simulink model "local"  (R2022a)
settings: Solver=VariableStepAuto  StartTime=0.0  StopTime=T_fin  FixedStep=0.0025  RelTol=1e-3
values from neighbouring files (symbols this model uses):
  A = A-B*k_leader    [project.m]
  Ad = [0 0 1 0 0 0; 1 0 0 0 0 0;0 1 0 0 0 0; 1 0 0 0 0 0; 0 0 0 0 0 0; 0 0 1 0 0 0]    [project.m]
  B = [0; -9.9453]    [project.m]
  C = [708.27 0]    [project.m]
  c = 5    [project.m]
  D_ = zeros(2,1)'    [project.m]
  F2 = place(A',-c*C',[-1 -2])'    [project.m]
  G = diag([1 0 0 0 1 0])    [project.m]
  K = inv(R)*B'*P    [project.m]
  L_leader = acker(A',C',[-1,-2])'    [project.m]
  X0 = [1/C(1) 1/800]'    [project.m]
settings Model: Creator=drurb  LastModifiedBy=Utente
settings DataIOCC: ReturnWorkspaceOutputs=off

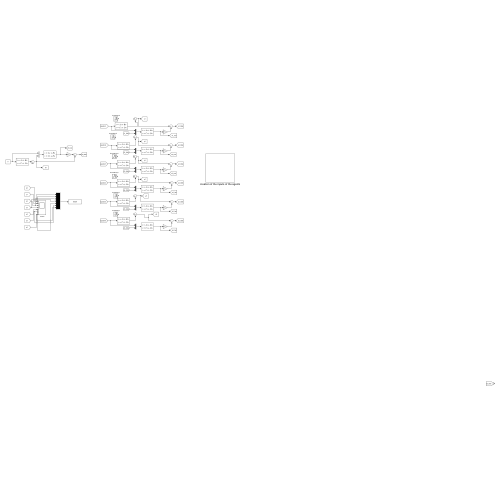
[thumbnail: Simulink's stored preview of the top-level diagram]
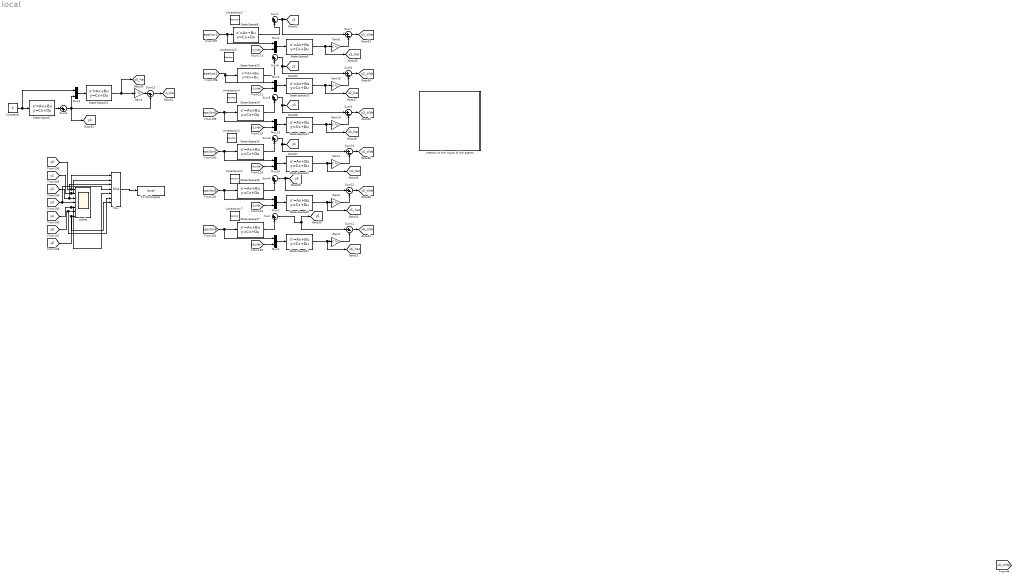
== system local ==
  Constant1 : Constant  Value=0
  Gain{1..5,13..14} (7 alike) : Gain  Gain=C  Multiplication=Matrix(K*u)
  Locale : Scope  NumInputPorts=7
  Mux : Mux  Inputs=7
  Mux{1..5,13..14} (7 alike) : Mux  Inputs=2
  State-Space{9..12,20..21} (6 alike) : StateSpace  A=A  B=[B*c*K -c*F2]  C=eye(2)  D=zeros(2,3)  InitialCondition=zeros(1,2)
  State-Space22 : StateSpace  A=A - L_leader*C  B=[B L_leader]  C=eye(2)  D=zeros(2,2)  InitialCondition=zeros(1,2)
  State-Space23 : StateSpace  A=A  B=B*c*K  C=C  D=D_  InitialCondition=[0 2/800]'
  State-Space24 : StateSpace  A=A  B=B*c*K  C=C  D=D_  InitialCondition=[-1/C(1) -1/800]
  State-Space25 : StateSpace  A=A  B=B*c*K  C=C  D=D_  InitialCondition=[3/C(1) -3/800]'
  State-Space26 : StateSpace  A=A  B=B*c*K  C=C  D=D_  InitialCondition=[2/C(1) 4/800]'
  State-Space27 : StateSpace  A=A  B=B*c*K  C=C  D=D_  InitialCondition=[-2/C(1) 0]'
  State-Space7 : StateSpace  A=A  B=B  C=C  D=0  InitialCondition=X0
  State-Space8 : StateSpace  A=A  B=B*c*K  C=C  D=D_  InitialCondition=[2/C(1) 1/800]'
  Sum{,1..6} (7 alike) : Sum  Inputs=|++
  Sum{7..12} (6 alike) : Sum  Inputs=|+-
  Sum13 : Sum  Inputs=|-+
  To Workspace : ToWorkspace  VariableName=local  SaveFormat=Timeseries  SampleTime=-1
  Uncertainty1 : RandomNumber  Mean=zeros(1,1)  Variance=0.1  Seed=1  SampleTime=0.1
  Uncertainty2 : RandomNumber  Seed=2  SampleTime=0.2
  Uncertainty3 : RandomNumber  Mean=zeros(1,1)  Variance=0.7  Seed=3  SampleTime=0.1
  Uncertainty4 : RandomNumber  Mean=zeros(1,1)  Variance=0.2  Seed=7  SampleTime=0.1
  Uncertainty5 : RandomNumber  Mean=zeros(1,1)  Variance=0.5  Seed=7  SampleTime=0.1
  Uncertainty7 : RandomNumber  Mean=zeros(1,1)  Variance=0.4  Seed=3  SampleTime=0.1
  creation of the inputs of the agents : Subsystem
  tag scope: x0_hat=global, x1_hat=global, x2_hat=global, x3_hat=global, x4_hat=global, x5_hat=global, x6_hat=global, y0=global, y0_tilde=global, y1=global, y1_tilde=global, y2=global, y2_tilde=global, y3=global, y3_tilde=global, y4=global, y4_tilde=global, y5=global, y5_tilde=global, y6=global, y6_tilde=global
  wires:
  State-Space11/1 -> [x3_hat], Gain14/1
  Gain1/1 -> Sum10/2
  [y1_tilde] -> Mux4/2
  Gain2/1 -> Sum11/2
  [epsilon4] -> State-Space25/1, Mux14/1
  Mux14/1 -> State-Space12/1
  Sum11/1 -> [y5_tilde]
  State-Space21/1 -> [x6_hat], Gain3/1
  Sum7/1 -> [y1_tilde]
  [y4_tilde] -> Mux14/2
  [epsilon2] -> State-Space23/1, Mux5/1
  Gain3/1 -> Sum12/2
  [epsilon5] -> State-Space26/1, Mux1/1
  State-Space9/1 -> Gain5/1, [x1_hat]
  Mux3/1 -> State-Space22/1
  [epsilon3] -> Mux13/1, State-Space24/1
  Sum12/1 -> [y6_tilde]
  [epsilon6] -> State-Space27/1, Mux2/1
  [epsilon1] -> Mux4/1, State-Space8/1
  Mux4/1 -> State-Space9/1
  [y5_tilde] -> Mux1/2
  [y3_tilde] -> Mux13/2
  Constant1/1 -> Mux3/1, State-Space7/1
  Sum10/1 -> [y4_tilde]
  [y3] -> Locale/4, Mux/4
  Mux2/1 -> State-Space21/1
  Gain4/1 -> Sum13/1
  Mux13/1 -> State-Space11/1
  Gain13/1 -> Sum8/2
  State-Space10/1 -> [x2_hat], Gain13/1
  Gain14/1 -> Sum9/2
  [y0] -> Mux/1, Locale/1
  [y1] -> Mux/2, Locale/2
  [y6] -> Mux/7, Locale/7
  [y6_tilde] -> Mux2/2
  Mux5/1 -> State-Space10/1
  State-Space20/1 -> [x5_hat], Gain2/1
  State-Space26/1 -> Sum4/2
  Mux1/1 -> State-Space20/1
  State-Space22/1 -> Gain4/1, [x0_hat]
  Sum9/1 -> [y3_tilde]
  Sum13/1 -> [y0_tilde]
  [y2_tilde] -> Mux5/2
  [y5] -> Locale/6, Mux/6
  State-Space12/1 -> [x4_hat], Gain1/1
  [y4] -> Mux/5, Locale/5
  Sum8/1 -> [y2_tilde]
  [y2] -> Locale/3, Mux/3
  Gain5/1 -> Sum7/2
  Mux/1 -> To Workspace/1
  State-Space27/1 -> Sum/2
  Sum/1 -> Sum12/1, [y6]
  Sum1/1 -> Sum7/1, [y1]
  State-Space8/1 -> Sum1/2
  State-Space7/1 -> Sum2/1
  Sum2/1 -> Sum13/2, [y0], Mux3/2
  State-Space25/1 -> Sum3/2
  Sum3/1 -> Sum10/1, [y4]
  Sum4/1 -> Sum11/1, [y5]
  Sum6/1 -> Sum8/1, [y2]
  State-Space23/1 -> Sum6/2
  Sum5/1 -> Sum9/1, [y3]
  State-Space24/1 -> Sum5/2

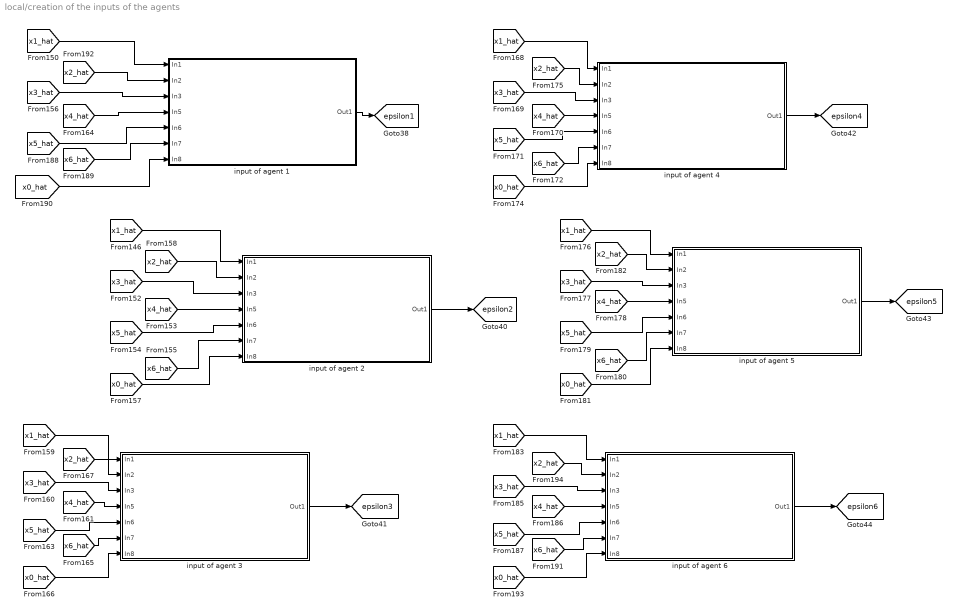
== system local/creation of the inputs of the agents ==
  input of agent 1 : Subsystem
  input of agent 2 : Subsystem
  input of agent 3 : Subsystem
  input of agent 4 : Subsystem
  input of agent 5 : Subsystem
  input of agent 6 : Subsystem
  tag scope: epsilon1=global, epsilon2=global, epsilon3=global, epsilon4=global, epsilon5=global, epsilon6=global
  wires:
  [x6_hat] -> input of agent 6/6(In7)
  input of agent 2/1(Out1) -> [epsilon2]
  [x0_hat] -> input of agent 3/7(In8)
  input of agent 6/1(Out1) -> [epsilon6]
  [x6_hat] -> input of agent 5/6(In7)
  [x2_hat] -> input of agent 5/2(In2)
  [x1_hat] -> input of agent 2/1(In1)
  [x1_hat] -> input of agent 4/1(In1)
  [x0_hat] -> input of agent 4/7(In8)
  [x5_hat] -> input of agent 1/5(In6)
  [x4_hat] -> input of agent 1/4(In5)
  [x4_hat] -> input of agent 5/4(In5)
  [x4_hat] -> input of agent 2/4(In5)
  input of agent 5/1(Out1) -> [epsilon5]
  [x3_hat] -> input of agent 6/3(In3)
  [x5_hat] -> input of agent 5/5(In6)
  [x5_hat] -> input of agent 3/5(In6)
  [x2_hat] -> input of agent 2/2(In2)
  [x4_hat] -> input of agent 6/4(In5)
  [x0_hat] -> input of agent 2/7(In8)
  [x5_hat] -> input of agent 6/5(In6)
  [x6_hat] -> input of agent 3/6(In7)
  [x1_hat] -> input of agent 5/1(In1)
  [x0_hat] -> input of agent 6/7(In8)
  [x3_hat] -> input of agent 1/3(In3)
  [x5_hat] -> input of agent 4/5(In6)
  [x3_hat] -> input of agent 3/3(In3)
  input of agent 4/1(Out1) -> [epsilon4]
  [x5_hat] -> input of agent 2/5(In6)
  [x1_hat] -> input of agent 1/1(In1)
  [x4_hat] -> input of agent 3/4(In5)
  [x4_hat] -> input of agent 4/4(In5)
  [x0_hat] -> input of agent 5/7(In8)
  [x1_hat] -> input of agent 6/1(In1)
  [x6_hat] -> input of agent 2/6(In7)
  [x2_hat] -> input of agent 6/2(In2)
  [x6_hat] -> input of agent 4/6(In7)
  [x2_hat] -> input of agent 1/2(In2)
  [x2_hat] -> input of agent 3/2(In2)
  [x3_hat] -> input of agent 4/3(In3)
  [x3_hat] -> input of agent 5/3(In3)
  [x0_hat] -> input of agent 1/7(In8)
  [x3_hat] -> input of agent 2/3(In3)
  [x1_hat] -> input of agent 3/1(In1)
  input of agent 3/1(Out1) -> [epsilon3]
  input of agent 1/1(Out1) -> [epsilon1]
  [x6_hat] -> input of agent 1/6(In7)
  [x2_hat] -> input of agent 4/2(In2)

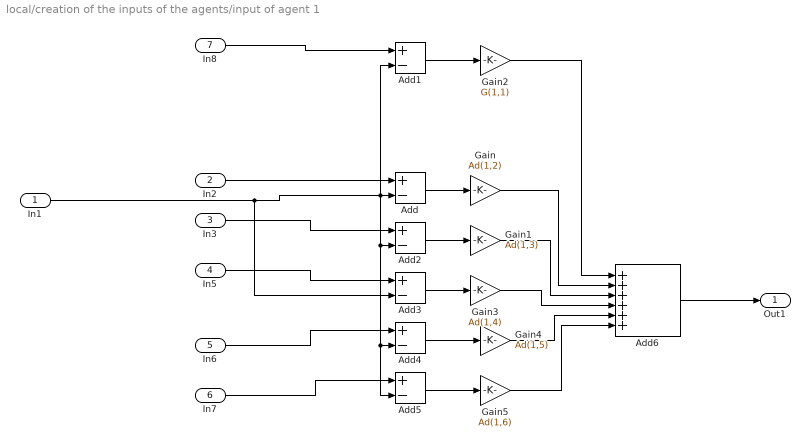
== system local/creation of the inputs of the agents/input of agent 1 ==
  In1 : Inport
  In2 : Inport  Port=2
  In3 : Inport  Port=3
  In5 : Inport  Port=4
  In6 : Inport  Port=5
  In7 : Inport  Port=6
  In8 : Inport  Port=7
  Add{,1..5} (6 alike) : Sum  Inputs=+-
  Add6 : Sum  Inputs=++++++
  Gain : Gain  Gain=Ad(1,2)
  Gain1 : Gain  Gain=Ad(1,3)
  Gain2 : Gain  Gain=G(1,1)
  Gain3 : Gain  Gain=Ad(1,4)
  Gain4 : Gain  Gain=Ad(1,5)
  Gain5 : Gain  Gain=Ad(1,6)
  Out1 : Outport
  wires:
  Add/1 -> Gain/1
  In1/1 -> Add3/2, Add5/2, Add4/2, Add2/2, Add/2, Add1/2
  In2/1 -> Add/1
  In8/1 -> Add1/1
  Add2/1 -> Gain1/1
  Add3/1 -> Gain3/1
  Add4/1 -> Gain4/1
  Add5/1 -> Gain5/1
  In3/1 -> Add2/1
  In5/1 -> Add3/1
  In6/1 -> Add4/1
  In7/1 -> Add5/1
  Gain/1 -> Add6/2
  Gain1/1 -> Add6/3
  Gain3/1 -> Add6/4
  Gain4/1 -> Add6/5
  Gain5/1 -> Add6/6
  Add1/1 -> Gain2/1
  Gain2/1 -> Add6/1
  Add6/1 -> Out1/1

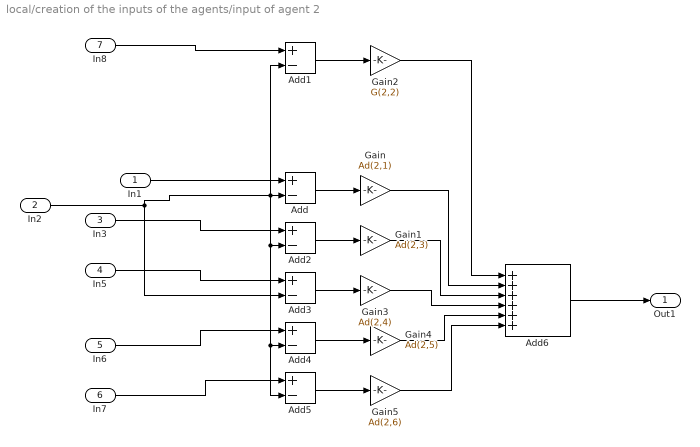
== system local/creation of the inputs of the agents/input of agent 2 ==
  In1 : Inport
  In2 : Inport  Port=2
  In3 : Inport  Port=3
  In5 : Inport  Port=4
  In6 : Inport  Port=5
  In7 : Inport  Port=6
  In8 : Inport  Port=7
  Add{,1..5} (6 alike) : Sum  Inputs=+-
  Add6 : Sum  Inputs=++++++
  Gain : Gain  Gain=Ad(2,1)
  Gain1 : Gain  Gain=Ad(2,3)
  Gain2 : Gain  Gain=G(2,2)
  Gain3 : Gain  Gain=Ad(2,4)
  Gain4 : Gain  Gain=Ad(2,5)
  Gain5 : Gain  Gain=Ad(2,6)
  Out1 : Outport
  wires:
  Add/1 -> Gain/1
  In2/1 -> Add3/2, Add5/2, Add4/2, Add2/2, Add/2, Add1/2
  In1/1 -> Add/1
  In8/1 -> Add1/1
  Add2/1 -> Gain1/1
  Add3/1 -> Gain3/1
  Add4/1 -> Gain4/1
  Add5/1 -> Gain5/1
  In3/1 -> Add2/1
  In5/1 -> Add3/1
  In6/1 -> Add4/1
  In7/1 -> Add5/1
  Gain/1 -> Add6/2
  Gain1/1 -> Add6/3
  Gain3/1 -> Add6/4
  Gain4/1 -> Add6/5
  Gain5/1 -> Add6/6
  Add1/1 -> Gain2/1
  Gain2/1 -> Add6/1
  Add6/1 -> Out1/1

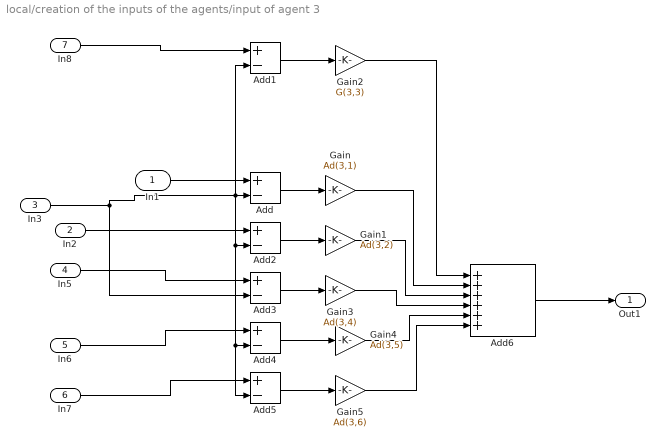
== system local/creation of the inputs of the agents/input of agent 3 ==
  In1 : Inport
  In2 : Inport  Port=2
  In3 : Inport  Port=3
  In5 : Inport  Port=4
  In6 : Inport  Port=5
  In7 : Inport  Port=6
  In8 : Inport  Port=7
  Add{,1..5} (6 alike) : Sum  Inputs=+-
  Add6 : Sum  Inputs=++++++
  Gain : Gain  Gain=Ad(3,1)
  Gain1 : Gain  Gain=Ad(3,2)
  Gain2 : Gain  Gain=G(3,3)
  Gain3 : Gain  Gain=Ad(3,4)
  Gain4 : Gain  Gain=Ad(3,5)
  Gain5 : Gain  Gain=Ad(3,6)
  Out1 : Outport
  wires:
  Add/1 -> Gain/1
  In3/1 -> Add3/2, Add5/2, Add4/2, Add2/2, Add/2, Add1/2
  In8/1 -> Add1/1
  Add2/1 -> Gain1/1
  Add3/1 -> Gain3/1
  Add4/1 -> Gain4/1
  Add5/1 -> Gain5/1
  In2/1 -> Add2/1
  In5/1 -> Add3/1
  In6/1 -> Add4/1
  In7/1 -> Add5/1
  Gain/1 -> Add6/2
  Gain1/1 -> Add6/3
  Gain3/1 -> Add6/4
  Gain4/1 -> Add6/5
  Gain5/1 -> Add6/6
  Add1/1 -> Gain2/1
  Gain2/1 -> Add6/1
  Add6/1 -> Out1/1
  In1/1 -> Add/1

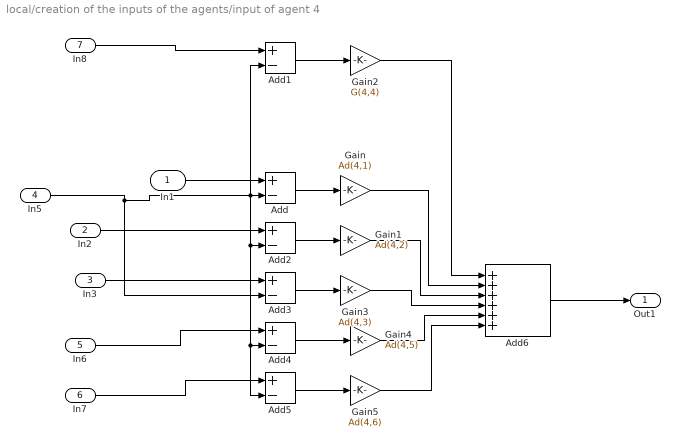
== system local/creation of the inputs of the agents/input of agent 4 ==
  In1 : Inport
  In2 : Inport  Port=2
  In3 : Inport  Port=3
  In5 : Inport  Port=4
  In6 : Inport  Port=5
  In7 : Inport  Port=6
  In8 : Inport  Port=7
  Add{,1..5} (6 alike) : Sum  Inputs=+-
  Add6 : Sum  Inputs=++++++
  Gain : Gain  Gain=Ad(4,1)
  Gain1 : Gain  Gain=Ad(4,2)
  Gain2 : Gain  Gain=G(4,4)
  Gain3 : Gain  Gain=Ad(4,3)
  Gain4 : Gain  Gain=Ad(4,5)
  Gain5 : Gain  Gain=Ad(4,6)
  Out1 : Outport
  wires:
  Add/1 -> Gain/1
  In5/1 -> Add3/2, Add5/2, Add4/2, Add2/2, Add/2, Add1/2
  In8/1 -> Add1/1
  Add2/1 -> Gain1/1
  Add3/1 -> Gain3/1
  Add4/1 -> Gain4/1
  Add5/1 -> Gain5/1
  In2/1 -> Add2/1
  In3/1 -> Add3/1
  In6/1 -> Add4/1
  In7/1 -> Add5/1
  Gain/1 -> Add6/2
  Gain1/1 -> Add6/3
  Gain3/1 -> Add6/4
  Gain4/1 -> Add6/5
  Gain5/1 -> Add6/6
  Add1/1 -> Gain2/1
  Gain2/1 -> Add6/1
  Add6/1 -> Out1/1
  In1/1 -> Add/1

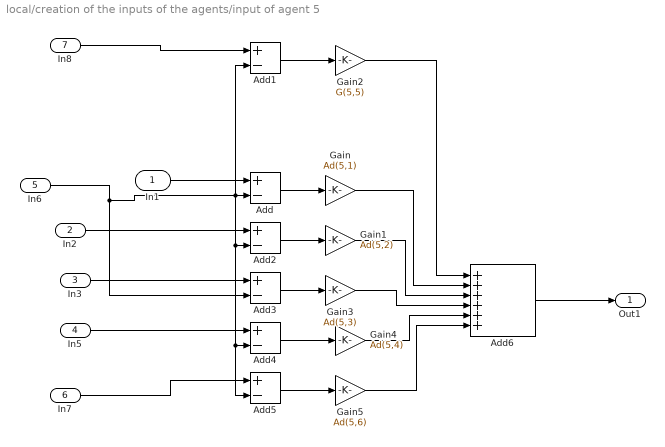
== system local/creation of the inputs of the agents/input of agent 5 ==
  In1 : Inport
  In2 : Inport  Port=2
  In3 : Inport  Port=3
  In5 : Inport  Port=4
  In6 : Inport  Port=5
  In7 : Inport  Port=6
  In8 : Inport  Port=7
  Add{,1..5} (6 alike) : Sum  Inputs=+-
  Add6 : Sum  Inputs=++++++
  Gain : Gain  Gain=Ad(5,1)
  Gain1 : Gain  Gain=Ad(5,2)
  Gain2 : Gain  Gain=G(5,5)
  Gain3 : Gain  Gain=Ad(5,3)
  Gain4 : Gain  Gain=Ad(5,4)
  Gain5 : Gain  Gain=Ad(5,6)
  Out1 : Outport
  wires:
  Add/1 -> Gain/1
  In6/1 -> Add3/2, Add5/2, Add4/2, Add2/2, Add/2, Add1/2
  In8/1 -> Add1/1
  Add2/1 -> Gain1/1
  Add3/1 -> Gain3/1
  Add4/1 -> Gain4/1
  Add5/1 -> Gain5/1
  In2/1 -> Add2/1
  In3/1 -> Add3/1
  In5/1 -> Add4/1
  In7/1 -> Add5/1
  Gain/1 -> Add6/2
  Gain1/1 -> Add6/3
  Gain3/1 -> Add6/4
  Gain4/1 -> Add6/5
  Gain5/1 -> Add6/6
  Add1/1 -> Gain2/1
  Gain2/1 -> Add6/1
  Add6/1 -> Out1/1
  In1/1 -> Add/1

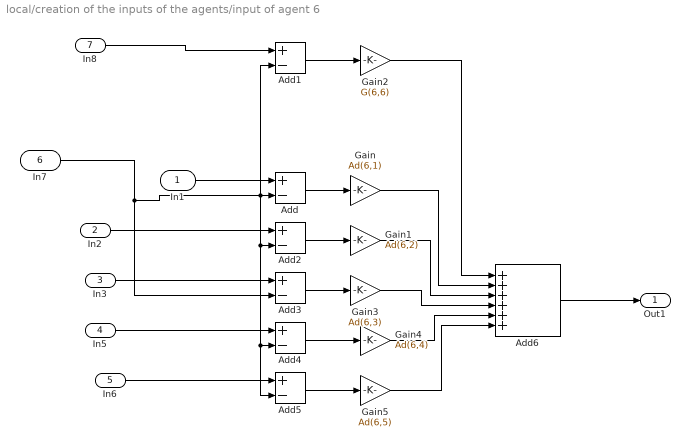
== system local/creation of the inputs of the agents/input of agent 6 ==
  In1 : Inport
  In2 : Inport  Port=2
  In3 : Inport  Port=3
  In5 : Inport  Port=4
  In6 : Inport  Port=5
  In7 : Inport  Port=6
  In8 : Inport  Port=7
  Add{,1..5} (6 alike) : Sum  Inputs=+-
  Add6 : Sum  Inputs=++++++
  Gain : Gain  Gain=Ad(6,1)
  Gain1 : Gain  Gain=Ad(6,2)
  Gain2 : Gain  Gain=G(6,6)
  Gain3 : Gain  Gain=Ad(6,3)
  Gain4 : Gain  Gain=Ad(6,4)
  Gain5 : Gain  Gain=Ad(6,5)
  Out1 : Outport
  wires:
  Add/1 -> Gain/1
  In7/1 -> Add3/2, Add5/2, Add4/2, Add2/2, Add/2, Add1/2
  In8/1 -> Add1/1
  Add2/1 -> Gain1/1
  Add3/1 -> Gain3/1
  Add4/1 -> Gain4/1
  Add5/1 -> Gain5/1
  In2/1 -> Add2/1
  In3/1 -> Add3/1
  In5/1 -> Add4/1
  In6/1 -> Add5/1
  Gain/1 -> Add6/2
  Gain1/1 -> Add6/3
  Gain3/1 -> Add6/4
  Gain4/1 -> Add6/5
  Gain5/1 -> Add6/6
  Add1/1 -> Gain2/1
  Gain2/1 -> Add6/1
  Add6/1 -> Out1/1
  In1/1 -> Add/1
